simulink model "bcSimPID"  (R2024a)
settings: Solver=FixedStepDiscrete  StartTime=0.0  StopTime=3.0  FixedStep=5e-6  MaxStep=1e-4  RelTol=1e-3
libraries: spsSeriesRLCBranchLib x3, spsDiodeLib x1, spsMosfetLib x1, simulink x1, spsPWMGeneratorDCDCLib x1, spsVoltageMeasurementLib x1, spsDCVoltageSourceLib x1, spspowerguiLib x1
settings Model: Creator=Dr. Javed  LastModifiedBy=ariellevy
settings SolverCC: AlgebraicLoopSolver=TrustRegion  PositivePriorityOrder=on
settings DataIOCC: ReturnWorkspaceOutputs=off
settings DebuggingCC: UnconnectedInputMsg=warning  UnconnectedOutputMsg=warning  UnconnectedLineMsg=warning  ArithmeticOperatorsInVariantConditions=warning
settings ModelReferenceCC: EnableRefExpFcnMdlSchedulingChecks=on
settings SFSimCC: SimUseLocalCustomCode=off  CustomCodeUndefinedFunction=UseInterfaceOnly
settings RTWCC: RTWUseLocalCustomCode=off  GPUComputeCapability=3.5
settings CodeAppCC: StateflowObjectComments=on
settings SimscapeCC: SimscapeNormalizeSystem=off

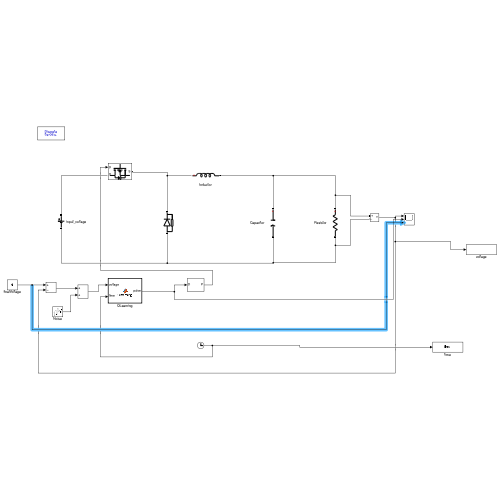
[thumbnail: Simulink's stored preview of the top-level diagram]
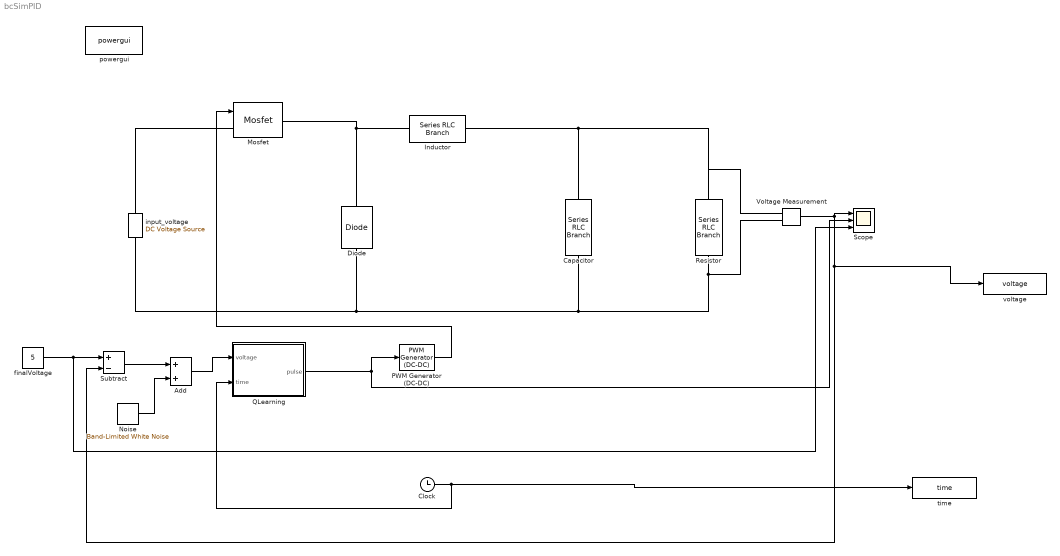
== system bcSimPID ==
  Add : Sum
  Capacitor : spsSeriesRLCBranchLib/Series RLC Branch  LConnTagsString=__new0  RConnTagsString=__new0  BranchType=C  Resistance=1  Inductance=100e-6  SetiL0=off  InitialCurrent=0  Capacitance=1000e-6  Setx0=off  InitialVoltage=0  Measurements=None
  Clock : Clock
  Diode : spsDiodeLib/Diode  Ron=0.001  Lon=0  Vf=0.8  IC=0  UseSnubber=0  Rs=500  Cs=250e-9  Measurements=off
  Inductor : spsSeriesRLCBranchLib/Series RLC Branch  LConnTagsString=__new0  RConnTagsString=__new0  BranchType=L  Resistance=1  Inductance=100e-6  SetiL0=off  InitialCurrent=0  Capacitance=1e-6  Setx0=off  InitialVoltage=0  Measurements=None
  Mosfet : spsMosfetLib/Mosfet  Ron=0.1  Lon=0  Rd=0.01  Vfd=0  IC=0  Rs=1e5  Cs=inf  Measurements=off
  Noise : simulink/Sources/Band-Limited White Noise  Cov=[0.00001]  Ts=5e-6  seed=[23341]
  PWM Generator (DC-DC) : spsPWMGeneratorDCDCLib/PWM Generator (DC-DC)  Fsw=10e3  Ts=5e-6
  QLearning : MATLAB Function  TreatAsAtomicUnit=on  SystemSampleTime=0.0001
  Resistor : spsSeriesRLCBranchLib/Series RLC Branch  LConnTagsString=__new0  RConnTagsString=__new0  BranchType=R  Resistance=10  Inductance=100e-6  SetiL0=off  InitialCurrent=0  Capacitance=1000e-6  Setx0=off  InitialVoltage=0  Measurements=None
  Scope : Scope  NumInputPorts=3
  Subtract : Sum  Inputs=+-
  Voltage Measurement : spsVoltageMeasurementLib/Voltage Measurement  PhasorSimulation=off  OutputType=Complex  PSBequivalent=0
  finalVoltage : Constant  Value=5
  input_voltage : spsDCVoltageSourceLib/DC Voltage Source  Amplitude=12  Measurements=None
  powergui : spspowerguiLib/powergui  Priority=1  SimulationMode=Discrete  SampleTime=5e-6  frequency=60  Iterations=50  frequencyindice=0  Pbase=100e6  ErrMax=1e-4  UnitsV=kV  UnitsW=MW  buscounter=0  FunctionMessages=off  echomessages=off  EnableUseOfTLC=off  CurrentSourceSwitches=off  DisableSnubberDevices=off  DisableRonSwitches=off  DisableVfSwitches=off  DisplayEquations=off  AutomaticDiscreteSolvers=off  SolverType=Tustin/Backward Euler (TBE)  Interpol=off  ExternalGateDelay=off  methode=off  Ts=100  x0status=blocks  SPID=on  SwTol=0  HookPort=off  NonlinearTolerance=1e-4  nMaxIteration=100  ContinueOnMaxIteration=off  RestoreLinks=warning  ResistiveCurrentMeasurement=off  Frange=[0:2:500]  Ylog=off  Xlog=on  ShowGrid=off  save=off  variable=ZData  structure=0  ZoomFFT=off  StartTime=0.0  cycles=1  DisplayStyle=1  fundamental=60  FreqAxis=off  MaxFrequency=1000  frequencyindicesteady=1  RmsSteady=1  display=off
  time : ToWorkspace  VariableName=time  SampleTime=-1
  voltage : ToWorkspace  VariableName=voltage  SampleTime=-1
  wires:
  Voltage Measurement/1 -> voltage/1, Subtract/2, Scope/1
  finalVoltage/1 -> Scope/3, Subtract/1
  PWM Generator (DC-DC)/1 -> Mosfet/1
  QLearning/1(pulse) -> Scope/2, PWM Generator (DC-DC)/1
  Clock/1 -> time/1, QLearning/2(time)
  Subtract/1 -> Add/1
  Add/1 -> QLearning/1(voltage)
  Noise/1 -> Add/2
  connections:
  Resistor/RConn1 -- Diode/LConn1 -- input_voltage/LConn1 -- Capacitor/RConn1 -- Voltage Measurement/LConn2
  Diode/RConn1 -- Mosfet/RConn1 -- Inductor/LConn1
  Capacitor/LConn1 -- Inductor/RConn1 -- Voltage Measurement/LConn1 -- Resistor/LConn1
  input_voltage/RConn1 -- Mosfet/LConn1

== matlab function bcSimPID/QLearning ==
  settings: updateMethod=DISCRETE
  data: voltage input; pulse output; time input
function pulse = Qlearning(voltage, time)

    % call extrinsic python function
    coder.extrinsic('py.PIDControllerBC.controller_call');

    % Call Python function and return result
    pulse = coder.nullcopy(zeros(1,1)); % no clue why, but this is need.
    pulse = double(py.PIDControllerBC.controller_call(voltage, time));
end
